simulink model "SolarSail"  (R2024a)
settings: Solver=ode3  StartTime=0.0  StopTime=2*24*60*60  FixedStep=30  MinStep=1  RelTol=1e-3
model workspace (MAT data in the model file):
  I_s = [344.15  0  0; 0  344.15  0; 0  0  688.24]
  LocalBodyOffset = [45 0 0]
undefined symbols (not defined in the file): IAU, juliandate, WMM2020
libraries: aerolibutil x15, matrix_library x14, simulink_extras x6, sharedtransform x5, aerolibtransform2 x4, aerolibconvert2 x4, aerolibatmos2 x1, aerolibsatdyn x1, aerolibobsolete x1, aerolibattitudesys x1, simulink x1, vrlib x1
(part 1 of 2)
settings Model: Creator=pierc  LastModifiedBy=pierc
settings SolverCC: InitialStep=1

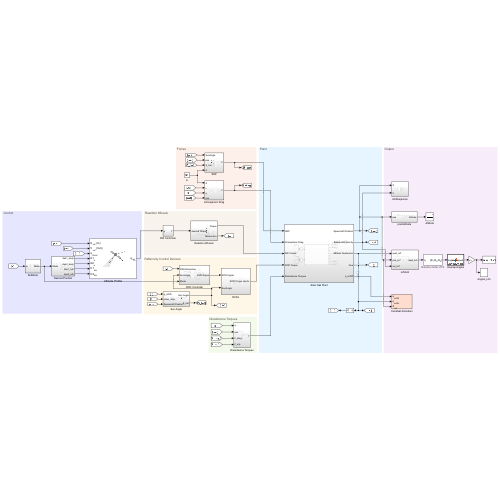
[thumbnail: Simulink's stored preview of the top-level diagram]
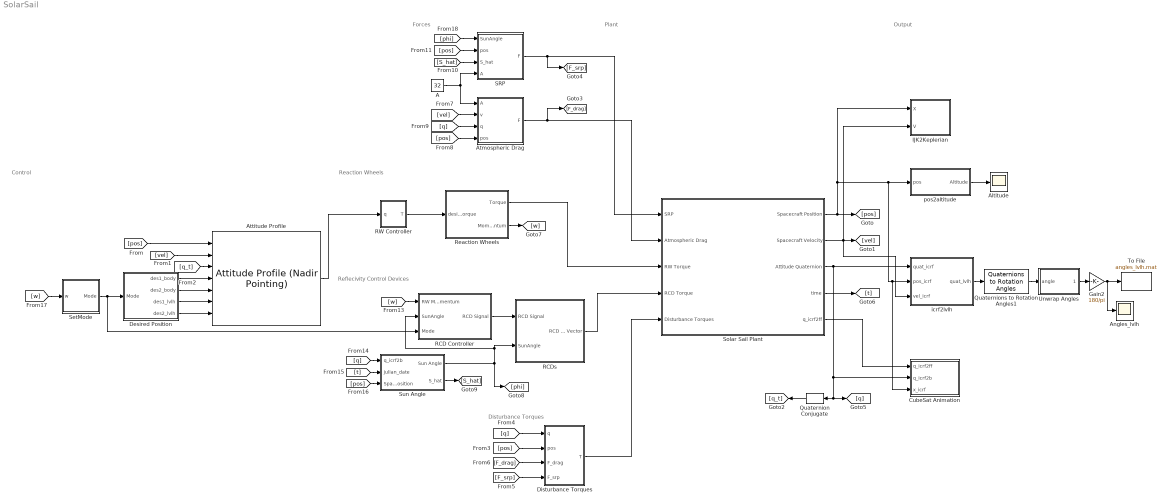
== system SolarSail ==
  note: Control
  note: Plant
  note: Reaction Wheels
  note: Disturbance Torques
  note: Forces
  note: Output
  note: Reflecivity Control Devices
  A : Constant  Value=32
  Altitude : Scope
  Angles_lvlh : Scope
  Atmospheric Drag : Subsystem
  "Attitude Profile " : aerolibsatdyn/Attitude Profile (Nadir Pointing)  outputError=on  outputFinalAttitude=off  portFrame=ICRF  pointingMode=Custom  celestialTarget=Sun  tunablePointing=off  primaryAlignmentSrc=Port  primaryAlignment=[0 0 1]  secondaryAlignmentSrc=Port  secondaryAlignment=[1 0 0]  constraintFrame=LVLH  primaryConstraintSrc=Port  primaryConstraint=[1 0 0]  secondaryConstraintSrc=Port  secondaryConstraint=[0 1 0]
  CubeSat Animation : Subsystem  mask(Simulink 3D Animation of CubeSat){enableVis=on, startDate=juliandate(2024, 7, 11, 2, 0, 0), visSampleTime=60, cubesatSize=2e5, showAntenna=on, antennaHeight=1e6, antennaHalfAngle=15}
      mask prompts: enableVis "spacecraft:cubesat:AnimEnableVis"; startDate "spacecraft:cubesat:StartDate"; visSampleTime "spacecraft:cubesat:AnimSampleTime"; cubesatSize "spacecraft:cubesat:MdlSize"; showAntenna "spacecraft:cubesat:ShowCone"; antennaHeight "spacecraft:cubesat:ConeHeight"; antennaHalfAngle "spacecraft:cubesat:ConeAngle"
      mask help: spacecraft:cubesat:VisBlockDesc
      settings: OpenFcn=|
      | if ~builtin('license','test','virtual_reality_toolbox')
      |     set_param(gcb, 'enableVis', 'off');
      | end
      | open_system(gcb,'mask');
      mask Callback enableVis:
      | if strcmp(get_param(gcb,'enableVis'), 'on')
      |     [licAvail, ~] = builtin('license','checkout','Virtual_Reality_Toolbox');
      |     if licAvail
      |         enable = repmat({'on'},7,1);
      |         set_param(gcb, 'Commented', 'off');
      |     else
      |         enable = repmat({'off'},7,1);
      |         set_param(gcb, 'Commented', 'on');
      |         set_param(gcb,'enableVis', 'off');
      |     end
      |     clear licAvail
      | else
      |     enable = repmat({'off'},7,1);
      |     set_param(gcb, 'Commented', 'on');
      | end
      | enable{1} = 'on';
      | set_param(gcb,'MaskEnables', enable);
      | clear enable
      mask Callback showAntenna:
      | if strcmp(get_param(gcb, 'enableVis'), 'on')
      |     enable = get_param(gcb,'MaskEnables');
      |     if strcmp(get_param(gcb, 'showAntenna'), 'off')
      |         enable(6:7) = {'off'};
      |     else
      |         enable(6:7) = {'on'};
      |     end
      |     set_param(gcb,'MaskEnables', enable);
      |     clear enable
      | end
      mask DialogControl enableVis Prompt: Enable visualization with Simulink 3D Animation
      mask DialogControl vrOpenBtn Prompt: spacecraft:cubesat:AnimOpenBtn
      mask DialogControl vrOpenBtn Callback:
      | if builtin('license','checkout','Virtual_Reality_Toolbox')
      |     vrmfunc('FnOpen',getSimulinkBlockHandle([gcb '/VR Sink']));
      | end
      mask DialogControl startDate Prompt: Start date [Julian date]:
      mask DialogControl startDate Tooltip: spacecraft:cubesat:StartDateTT
      mask DialogControl visSampleTime Prompt: Animation refresh rate:
      mask DialogControl visSampleTime Tooltip: spacecraft:cubesat:AnimSampleTimeTT
      mask DialogControl cubesatSize Prompt: CubeSat display size [m]:
      mask DialogControl cubesatSize Tooltip: spacecraft:cubesat:MdlSizeTT
      mask DialogControl Container3 Prompt: spacecraft:cubesat:AntennaPropArea
      mask DialogControl showAntenna Prompt: Show antenna cone in animation
      mask DialogControl showAntenna Tooltip: spacecraft:cubesat:ShowConeTT
      mask DialogControl antennaHeight Prompt: Antenna cone height [m]:
      mask DialogControl antennaHeight Tooltip: spacecraft:cubesat:ConeHeightTT
      mask DialogControl antennaHalfAngle Prompt: Antenna cone half angle [deg]:
      mask DialogControl antennaHalfAngle Tooltip: spacecraft:cubesat:ConeAngleTT
      mask Display:
      | port_label('input', 3, 'X_{icrf}','texmode','on')
      | port_label('input', 2, 'q_{icrf2b}','texmode','on')
      | port_label('input', 1, 'q_{icrf2ff}','texmode','on')
  Desired Position : Subsystem
  Disturbance Torques : Subsystem
  Gain2 : Gain  Gain=180/pi
  IJK2Keplerian : Subsystem
  Quaternion Conjugate : aerolibutil/Quaternion Conjugate
  Quaternions to Rotation Angles1 : sharedtransform/Quaternions to Rotation Angles  rotationOrder=ZYX  aMode=aMode
  RCD Controller : Subsystem
  RCDs : Subsystem
  RW Controller : Subsystem
  Reaction Wheels : Subsystem
  SRP : Subsystem
  SetMode : Subsystem
  Solar Sail Plant : Subsystem
  Sun Angle : Subsystem
  To File : ToFile  Filename=angles_lvlh.mat  MatrixName=angles_lvlh  SaveFormat=Timeseries
      settings: Decimation=2
  Unwrap Angles : MATLAB Function  TreatAsAtomicUnit=on  SystemSampleTime=30
  icrf2lvlh : Subsystem
  pos2altitude : Subsystem
  wires:
  Solar Sail Plant/1(Spacecraft Position) -> icrf2lvlh/2(pos_icrf), CubeSat Animation/3(x_icrf), pos2altitude/1(pos), IJK2Keplerian/1(X), [pos]
  Solar Sail Plant/3(Attitude Quaternion) -> icrf2lvlh/1(quat_icrf), [q], Quaternion Conjugate/1, CubeSat Animation/2(q_icrf2b)
  Solar Sail Plant/5(q_icrf2ff) -> CubeSat Animation/1(q_icrf2ff)
  Gain2/1 -> To File/1, Angles_lvlh/1
  [pos] -> "Attitude Profile "/1
  Solar Sail Plant/2(Spacecraft Velocity) -> IJK2Keplerian/2(V), [vel], icrf2lvlh/3(vel_icrf)
  Quaternion Conjugate/1 -> [q_t]
  [q_t] -> "Attitude Profile "/3
  icrf2lvlh/1(quat_lvlh) -> Quaternions to Rotation Angles1/1
  Desired Position/4(des2_lvlh) -> "Attitude Profile "/7
  "Attitude Profile "/1 -> RW Controller/1(q)
  Desired Position/1(des1_body) -> "Attitude Profile "/4
  Desired Position/2(des2_body) -> "Attitude Profile "/5
  Solar Sail Plant/4(time) -> [t]
  [vel] -> "Attitude Profile "/2
  RW Controller/1(T) -> Reaction Wheels/1(desired Torque)
  Reaction Wheels/1(Torque) -> Solar Sail Plant/3(RW Torque)
  pos2altitude/1(Altitude) -> Altitude/1
  [pos] -> Disturbance Torques/2(pos)
  [q] -> Disturbance Torques/1(q)
  Disturbance Torques/1(T) -> Solar Sail Plant/5(Disturbance Torques)
  [F_drag] -> Disturbance Torques/3(F_drag)
  [vel] -> Atmospheric Drag/2(v)
  [pos] -> Atmospheric Drag/4(pos)
  [q] -> Atmospheric Drag/3(q)
  Atmospheric Drag/1(F) -> [F_drag], Solar Sail Plant/2(Atmospheric Drag)
  [phi] -> SRP/1(SunAngle)
  A/1 -> Atmospheric Drag/1(A), SRP/4(A)
  SRP/1(F) -> [F_srp], Solar Sail Plant/1(SRP)
  [pos] -> Sun Angle/3(Spacecraft Position)
  [t] -> Sun Angle/2(julian_date)
  [q] -> Sun Angle/1(q_icrf2b)
  RCD Controller/1(RCD Signal) -> RCDs/1(RCD Signal)
  Sun Angle/1(Sun Angle) -> [phi], RCD Controller/2(SunAngle), RCDs/2(SunAngle)
  RCDs/1(RCD Torque Vector) -> Solar Sail Plant/4(RCD Torque)
  SetMode/1(Mode) -> RCD Controller/3(Mode), Desired Position/1(Mode)
  [w] -> RCD Controller/1(RW Momentum)
  Reaction Wheels/2(Momentum) -> [w]
  [w] -> SetMode/1(w)
  Desired Position/3(des1_lvlh) -> "Attitude Profile "/6
  Quaternions to Rotation Angles1/1 -> Unwrap Angles/1(angle)
  Unwrap Angles/1(unwrapped) -> Gain2/1
  [pos] -> SRP/2(pos)
  [F_srp] -> Disturbance Torques/4(F_srp)
  Sun Angle/2(S_hat) -> [S_hat]
  [S_hat] -> SRP/3(S_hat)

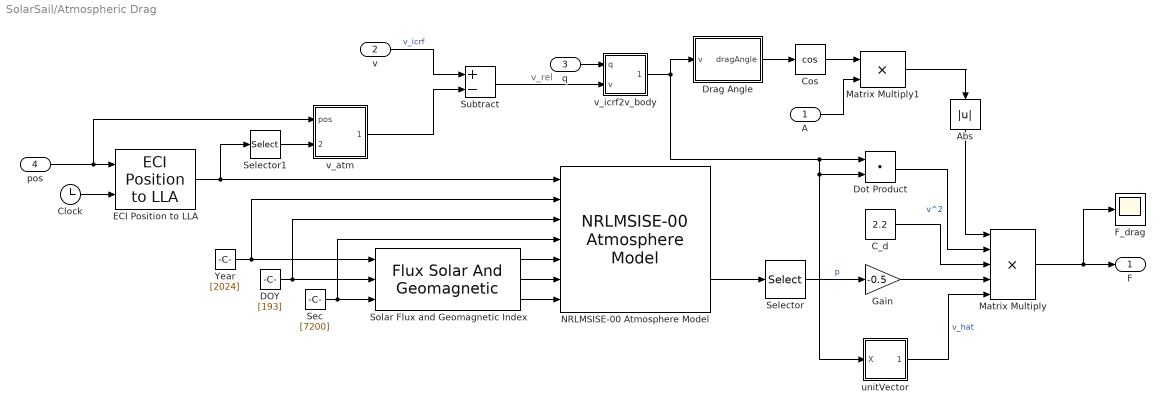
== system SolarSail/Atmospheric Drag ==
  note: v_rel
  A : Inport
  v : Inport  Port=2
  q : Inport  Port=3
  pos : Inport  Port=4
  Abs : Abs  SaturateOnIntegerOverflow=off
  C_d : Constant  Value=2.2
  Clock : Clock
  Cos : Trigonometry  Operator=cos
  DOY : Constant  Value=[193]
  Dot Product : DotProduct  OutDataTypeStr=Inherit: Inherit via internal rule
  Drag Angle : Subsystem
  ECI Position to LLA : aerolibtransform2/ECI Position to LLA  red=IAU-2000/2006  year=2024  month=July  day=11  hour=2  min=0  sec=0  deltaT=Sec  errorflag=Error  extraparamflag=off  eunits=Metric (MKS)  earthmodel=WGS84  flat=1/298.257223563  eqradius=6378137
      settings: AttributesFormatString=%<red>
  F_drag : Scope
  Gain : Gain  Gain=-0.5
  Matrix Multiply : Product  Inputs=5
  Matrix Multiply1 : Product
  NRLMSISE-00 Atmosphere Model : aerolibatmos2/NRLMSISE-00 Atmosphere Model  units=Metric (MKS)  lst_input=off  flux_ap_input=on  flags_input=Internal  flags=ones(1,23)  oxygen_in=on  action=Warning
  Sec : Constant  Value=[7200]
  Selector : Selector  InputPortWidth=9  IndexOptions=Index vector (dialog)  Indices=[6]  OutputSizes=1
  Selector1 : Selector  InputPortWidth=3  IndexOptions=Index vector (dialog)  Indices=[1]  OutputSizes=1
  Solar Flux and Geomagnetic Index : FluxSolarAndGeomagnetic
  Subtract : Sum  Inputs=+-
  Year : Constant  Value=[2024]
  unitVector : Subsystem
  v_atm : Subsystem
  v_icrf2v_body : Subsystem
  F : Outport
  wires:
  NRLMSISE-00 Atmosphere Model/2 -> Selector/1
  ECI Position to LLA/1 -> Selector1/1, NRLMSISE-00 Atmosphere Model/1
  pos/1 -> v_atm/1(pos), ECI Position to LLA/1
  DOY/1 -> NRLMSISE-00 Atmosphere Model/3, Solar Flux and Geomagnetic Index/2
  Solar Flux and Geomagnetic Index/3 -> NRLMSISE-00 Atmosphere Model/7
  Solar Flux and Geomagnetic Index/2 -> NRLMSISE-00 Atmosphere Model/6
  Clock/1 -> ECI Position to LLA/2
  Solar Flux and Geomagnetic Index/1 -> NRLMSISE-00 Atmosphere Model/5
  Gain/1 -> Matrix Multiply/4
  Selector/1 -> Gain/1  "p"
  Cos/1 -> Matrix Multiply1/1
  Drag Angle/1(dragAngle) -> Cos/1
  C_d/1 -> Matrix Multiply/3
  Matrix Multiply1/1 -> Abs/1
  Year/1 -> NRLMSISE-00 Atmosphere Model/2, Solar Flux and Geomagnetic Index/1
  Sec/1 -> NRLMSISE-00 Atmosphere Model/4, Solar Flux and Geomagnetic Index/3
  A/1 -> Matrix Multiply1/2
  Dot Product/1 -> Matrix Multiply/2  "v^2"
  Selector1/1 -> v_atm/2(latitude)
  v_atm/1(v_atm) -> Subtract/2
  Subtract/1 -> v_icrf2v_body/2(v)
  v/1 -> Subtract/1  "v_icrf"
  v_icrf2v_body/1(v_body) -> unitVector/1(X), Dot Product/2, Dot Product/1, Drag Angle/1(v)
  q/1 -> v_icrf2v_body/1(q)
  Matrix Multiply/1 -> F_drag/1, F/1
  Abs/1 -> Matrix Multiply/1
  unitVector/1(X_hat) -> Matrix Multiply/5  "v_hat"

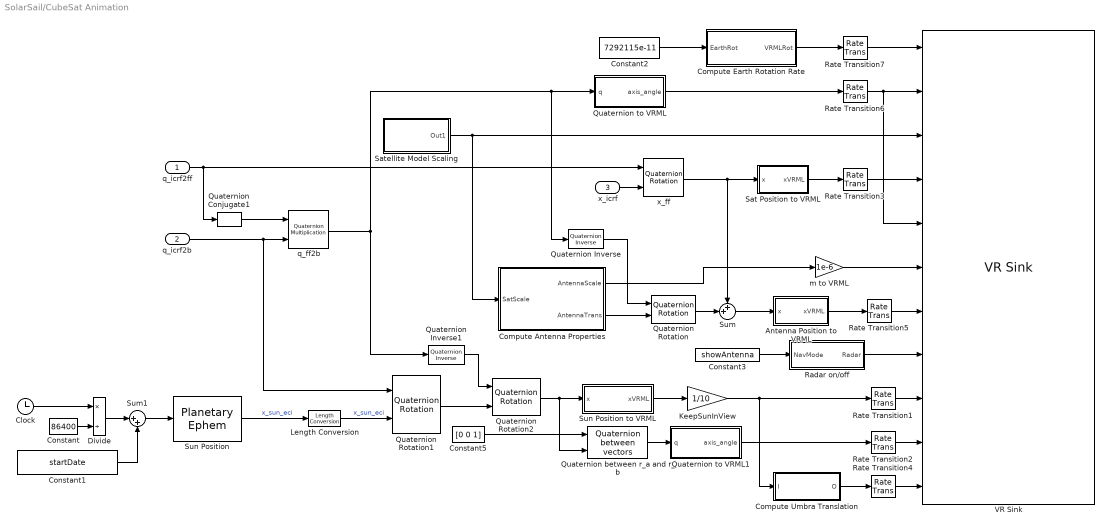
== system SolarSail/CubeSat Animation ==
  q_icrf2ff : Inport  PortDimensions=4
  q_icrf2b : Inport  Port=2  PortDimensions=4
  x_icrf : Inport  Port=3  PortDimensions=3
  Antenna Position to VRML : Subsystem
  Clock : Clock
  Compute Antenna Properties : Subsystem
  Compute Earth Rotation Rate : Subsystem
  Compute Umbra Translation : Subsystem
  Constant : Constant  Value=86400
  Constant1 : Constant  Value=startDate  SampleTime=visSampleTime
  Constant2 : Constant  Value=7292115e-11
  Constant3 : Constant  Value=showAntenna
  Constant5 : Constant  Value=[0 0 1]
  Divide : Product  Inputs=*/
  KeepSunInView : Gain  Gain=1/10
  Length Conversion : aerolibconvert2/Length Conversion  IU=km  OU=m
  Quaternion Conjugate1 : aerolibutil/Quaternion Conjugate
  Quaternion Inverse : aerolibutil/Quaternion Inverse
  Quaternion Inverse1 : aerolibutil/Quaternion Inverse
  Quaternion Rotation : aerolibutil/Quaternion Rotation
  Quaternion Rotation1 : aerolibutil/Quaternion Rotation
  Quaternion Rotation2 : aerolibutil/Quaternion Rotation
  Quaternion between r_a and r_b : aerolibattitudesys/Quaternion between vectors
  Quaternion to VRML : Subsystem
  Quaternion to VRML1 : Subsystem
  Radar on/off : Subsystem
  Rate Transition{1..7} (7 alike) : RateTransition
  Sat Position to VRML : Subsystem
  Satellite Model Scaling : Subsystem
  Sum : Sum  Inputs=++|
  Sum1 : Sum  Inputs=|++
  Sun Position : PlanetaryEphem  ephemerisModel=DE421  target=Sun  outputVelocity=off
  Sun Position to VRML : Subsystem
  VR Sink : vrlib/VR Sink  InstantiateOnLoad=on  SampleTime=visSampleTime  ViewEnable=on  RemoteChange=off  RemoteView=off  FieldsWritten=Earth.rotation.4.1.1.double#Satellite.rotation.4.1.1.double#Satellite.scale.3.1.1.double#Satellite.translation.3.1.1.double#AntennaCone.rotation.4.1.1.double#AntennaCone.scale.3.1.1.double#AntennaCone.translation.3.1.1.double#AntennaMaterial.transparency.1.1.1.double#Sun.translation.3.1.1.double#Umbra.rotation.4.1.1.double#Umbra.translation.3.1.1.double  WorldFileName=cubesatAnim.wrl  WorldDescription=CubeSat Orbit Animation  AutoView=off  VideoDimensions=[]  AllowVariableSize=off
  m to VRML : Gain  Gain=1e-6
  q_ff2b : aerolibutil/Quaternion Multiplication
  x_ff : aerolibutil/Quaternion Rotation
  wires:
  Quaternion to VRML1/1(axis_angle) -> Rate Transition2/1
  Quaternion between r_a and r_b/1 -> Quaternion to VRML1/1(q)
  Constant2/1 -> Compute Earth Rotation Rate/1(EarthRot)
  Compute Antenna Properties/1(AntennaScale) -> m to VRML/1
  Quaternion to VRML/1(axis_angle) -> Rate Transition6/1
  Compute Umbra Translation/1(O) -> Rate Transition4/1
  q_icrf2b/1 -> Quaternion Rotation1/1, q_ff2b/2
  Quaternion Rotation2/1 -> Sun Position to VRML/1(x), Quaternion between r_a and r_b/2
  Constant5/1 -> Quaternion between r_a and r_b/1
  KeepSunInView/1 -> Compute Umbra Translation/1(I), Rate Transition1/1
  Sun Position to VRML/1(xVRML) -> KeepSunInView/1
  Sat Position to VRML/1(xVRML) -> Rate Transition3/1
  Compute Antenna Properties/2(AntennaTrans) -> Quaternion Rotation/2
  Satellite Model Scaling/1(Out1) -> VR Sink/3, Compute Antenna Properties/1(SatScale)
  Constant3/1 -> Radar on/off/1(NavMode)
  q_ff2b/1 -> Quaternion Inverse/1, Quaternion to VRML/1(q), Quaternion Inverse1/1
  Quaternion Rotation1/1 -> Quaternion Rotation2/2
  Compute Earth Rotation Rate/1(VRMLRot) -> Rate Transition7/1
  Antenna Position to VRML/1(xVRML) -> Rate Transition5/1
  Quaternion Inverse/1 -> Quaternion Rotation/1
  x_ff/1 -> Sum/1, Sat Position to VRML/1(x)
  Quaternion Rotation/1 -> Sum/2
  Sum/1 -> Antenna Position to VRML/1(x)
  Quaternion Inverse1/1 -> Quaternion Rotation2/1
  Rate Transition4/1 -> VR Sink/11
  Rate Transition2/1 -> VR Sink/10
  Rate Transition1/1 -> VR Sink/9
  Rate Transition5/1 -> VR Sink/7
  m to VRML/1 -> VR Sink/6
  Rate Transition3/1 -> VR Sink/4
  Rate Transition7/1 -> VR Sink/1
  Rate Transition6/1 -> VR Sink/5, VR Sink/2
  Constant1/1 -> Sum1/2
  Divide/1 -> Sum1/1
  Constant/1 -> Divide/2
  Sun Position/1 -> Length Conversion/1  "x_sun_eci"
  Clock/1 -> Divide/1
  Length Conversion/1 -> Quaternion Rotation1/2  "x_sun_eci"
  Sum1/1 -> Sun Position/1
  Radar on/off/1(Radar) -> VR Sink/8
  Quaternion Conjugate1/1 -> q_ff2b/1
  q_icrf2ff/1 -> Quaternion Conjugate1/1, x_ff/1
  x_icrf/1 -> x_ff/2

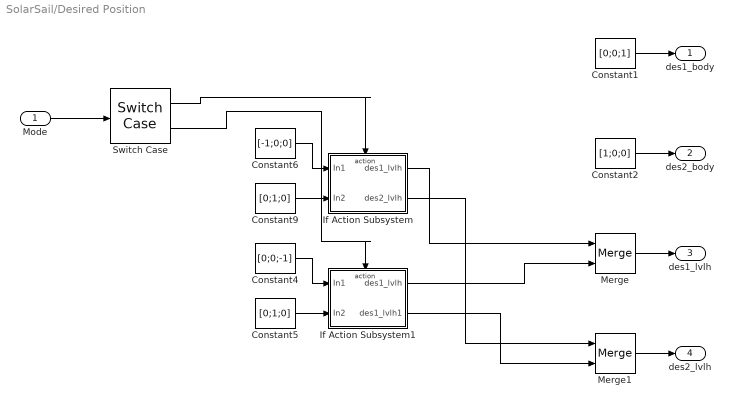
== system SolarSail/Desired Position ==
  Mode : Inport
  Constant1 : Constant  Value=[0;0;1]
  Constant2 : Constant  Value=[1;0;0]
  Constant4 : Constant  Value=[0;0;-1]
  Constant5 : Constant  Value=[0;1;0]
  Constant6 : Constant  Value=[-1;0;0]
  Constant9 : Constant  Value=[0;1;0]
  If Action Subsystem : Subsystem  TreatAsAtomicUnit=on
  If Action Subsystem1 : Subsystem  TreatAsAtomicUnit=on
  Merge : Merge
  Merge1 : Merge
  Switch Case : SwitchCase  CaseConditions={0,1}  ShowDefaultCase=off
  des1_body : Outport
  des2_body : Outport  Port=2
  des1_lvlh : Outport  Port=3
  des2_lvlh : Outport  Port=4
  wires:
  Constant1/1 -> des1_body/1
  Constant2/1 -> des2_body/1
  Mode/1 -> Switch Case/1
  Switch Case/1 -> If Action Subsystem/Action
  Constant6/1 -> If Action Subsystem/1(In1)
  Constant9/1 -> If Action Subsystem/2(In2)
  Switch Case/2 -> If Action Subsystem1/Action
  Constant4/1 -> If Action Subsystem1/1(In1)
  Constant5/1 -> If Action Subsystem1/2(In2)
  Merge/1 -> des1_lvlh/1
  Merge1/1 -> des2_lvlh/1
  If Action Subsystem/1(des1_lvlh) -> Merge/1
  If Action Subsystem1/1(des1_lvlh) -> Merge/2
  If Action Subsystem/2(des2_lvlh) -> Merge1/1
  If Action Subsystem1/2(des1_lvlh1) -> Merge1/2

== system SolarSail/Disturbance Torques ==
  q : Inport
  pos : Inport  Port=2
  F_drag : Inport  Port=3
  F_srp : Inport  Port=4
  Add : Sum  Inputs=+++
  Atmospheric Drag Torque : Subsystem
  Magnetic Field Torque : Subsystem
  SRP Torque : Subsystem
  T : Outport
  wires:
  pos/1 -> Magnetic Field Torque/1(pos)
  q/1 -> Magnetic Field Torque/2(q)
  Add/1 -> T/1  "T"
  F_drag/1 -> Atmospheric Drag Torque/1(F_drag)
  Atmospheric Drag Torque/1(T) -> Add/2
  SRP Torque/1(T) -> Add/1
  Magnetic Field Torque/1(T) -> Add/3
  F_srp/1 -> SRP Torque/1(F_srp)

== system SolarSail/IJK2Keplerian ==
  X : Inport
  V : Inport  Port=2
  Bus Creator : BusCreator  Inputs=6
  MATLAB Function : MATLAB Function  TreatAsAtomicUnit=on
  To Workspace : ToWorkspace  VariableName=OrbitalElements  SaveFormat=Timeseries  SampleTime=-1
  wires:
  X/1 -> MATLAB Function/1(r_ijk)
  V/1 -> MATLAB Function/2(v_ijk)
  MATLAB Function/1(a) -> Bus Creator/1
  MATLAB Function/2(ecc) -> Bus Creator/2
  MATLAB Function/3(incl) -> Bus Creator/3
  MATLAB Function/4(RAAN) -> Bus Creator/4
  MATLAB Function/5(argp) -> Bus Creator/5
  MATLAB Function/6(nu) -> Bus Creator/6
  Bus Creator/1 -> To Workspace/1

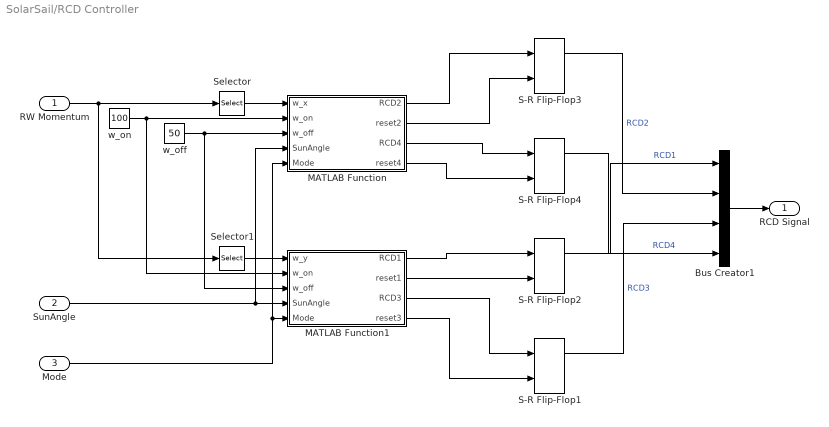
== system SolarSail/RCD Controller ==
  RW Momentum : Inport
  SunAngle : Inport  Port=2
  Mode : Inport  Port=3
  Bus Creator1 : BusCreator  Inputs=4
  MATLAB Function : MATLAB Function  TreatAsAtomicUnit=on
  MATLAB Function1 : MATLAB Function  TreatAsAtomicUnit=on
  S-R Flip-Flop{1..4} (4 alike) : simulink_extras/Flip Flops/S-R Flip-Flop  initial_condition=0
  Selector : Selector  InputPortWidth=3  IndexOptions=Index vector (dialog)  Indices=[1]  OutputSizes=1
  Selector1 : Selector  InputPortWidth=3  IndexOptions=Index vector (dialog)  Indices=[2]  OutputSizes=1
  w_off : Constant  Value=50
  w_on : Constant  Value=100
  RCD Signal : Outport
  wires:
  Bus Creator1/1 -> RCD Signal/1
  MATLAB Function1/1(RCD1) -> S-R Flip-Flop2/1
  MATLAB Function1/2(reset1) -> S-R Flip-Flop2/2
  MATLAB Function1/3(RCD3) -> S-R Flip-Flop1/1
  MATLAB Function1/4(reset3) -> S-R Flip-Flop1/2
  S-R Flip-Flop1/1 -> Bus Creator1/3  "RCD3"
  S-R Flip-Flop2/1 -> Bus Creator1/1  "RCD1"
  w_off/1 -> MATLAB Function1/3(w_off), MATLAB Function/3(w_off)
  w_on/1 -> MATLAB Function1/2(w_on), MATLAB Function/2(w_on)
  MATLAB Function/1(RCD2) -> S-R Flip-Flop3/1
  MATLAB Function/2(reset2) -> S-R Flip-Flop3/2
  MATLAB Function/3(RCD4) -> S-R Flip-Flop4/1
  MATLAB Function/4(reset4) -> S-R Flip-Flop4/2
  S-R Flip-Flop4/1 -> Bus Creator1/4  "RCD4"
  S-R Flip-Flop3/1 -> Bus Creator1/2  "RCD2"
  Selector/1 -> MATLAB Function/1(w_x)
  RW Momentum/1 -> Selector/1, Selector1/1
  Selector1/1 -> MATLAB Function1/1(w_y)
  SunAngle/1 -> MATLAB Function/4(SunAngle), MATLAB Function1/4(SunAngle)
  Mode/1 -> MATLAB Function/5(Mode), MATLAB Function1/5(Mode)

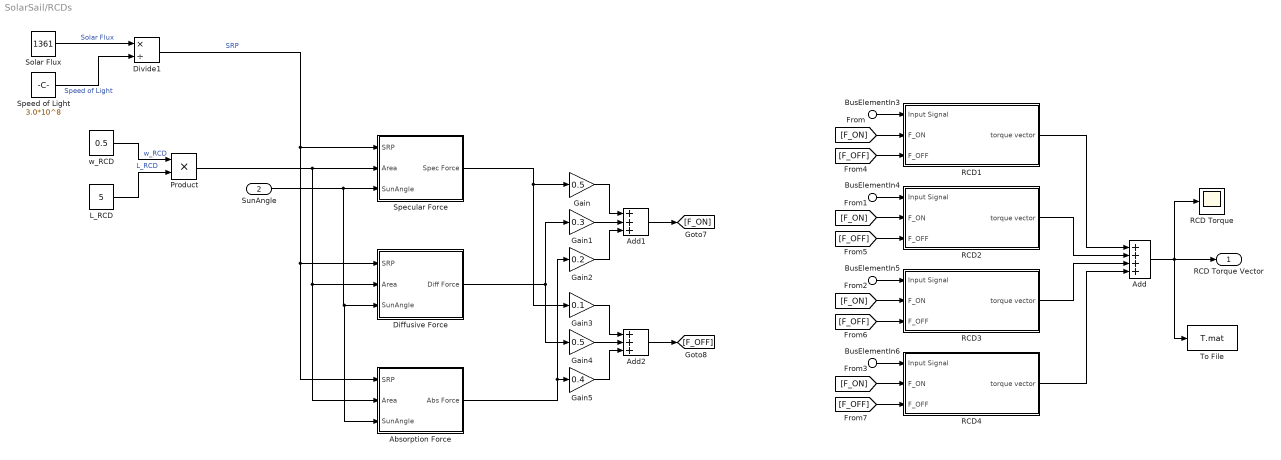
== system SolarSail/RCDs ==
  BusElementIn3 : Inport  PortName=RCD Signal  Element=RCD1
  BusElementIn4 : Inport  PortName=RCD Signal  Element=RCD2
  BusElementIn5 : Inport  PortName=RCD Signal  Element=RCD3
  BusElementIn6 : Inport  PortName=RCD Signal  Element=RCD4
  SunAngle : Inport  Port=2
  Absorption Force : Subsystem
  Add : Sum  Inputs=++++
  Add1 : Sum  Inputs=+++
  Add2 : Sum  Inputs=+++
  Diffusive Force : Subsystem
  Divide1 : Product  Inputs=*/
  Gain : Gain  Gain=0.5
  Gain1 : Gain  Gain=0.3
  Gain2 : Gain  Gain=0.2
  Gain3 : Gain  Gain=0.1
  Gain4 : Gain  Gain=0.5
  Gain5 : Gain  Gain=0.4
  L_RCD : Constant  Value=5
  Product : Product
  RCD Torque : Scope
  RCD1 : Subsystem
  RCD2 : Subsystem
  RCD3 : Subsystem
  RCD4 : Subsystem
  Solar Flux : Constant  Value=1361
  Specular Force : Subsystem
  Speed of Light : Constant  Value=3.0*10^8
  To File : ToFile  Filename=T.mat  MatrixName=T  SaveFormat=Timeseries
      settings: Decimation=2
  w_RCD : Constant  Value=0.5
  RCD Torque Vector : Outport
  wires:
  RCD2/1(torque vector) -> Add/2
  RCD1/1(torque vector) -> Add/1
  RCD4/1(torque vector) -> Add/4
  RCD3/1(torque vector) -> Add/3
  Add/1 -> To File/1, RCD Torque/1, RCD Torque Vector/1
  BusElementIn3/1 -> RCD1/1(Input Signal)
  BusElementIn4/1 -> RCD2/1(Input Signal)
  BusElementIn5/1 -> RCD3/1(Input Signal)
  [F_ON] -> RCD1/2(F_ON)
  [F_ON] -> RCD2/2(F_ON)
  [F_ON] -> RCD3/2(F_ON)
  [F_ON] -> RCD4/2(F_ON)
  [F_OFF] -> RCD1/3(F_OFF)
  [F_OFF] -> RCD2/3(F_OFF)
  [F_OFF] -> RCD3/3(F_OFF)
  [F_OFF] -> RCD4/3(F_OFF)
  BusElementIn6/1 -> RCD4/1(Input Signal)
  Speed of Light/1 -> Divide1/2  "Speed of Light"
  Solar Flux/1 -> Divide1/1  "Solar Flux"
  L_RCD/1 -> Product/2  "L_RCD"
  Divide1/1 -> Absorption Force/1(SRP), Diffusive Force/1(SRP), Specular Force/1(SRP)  "SRP"
  w_RCD/1 -> Product/1  "w_RCD"
  Add1/1 -> [F_ON]
  Gain/1 -> Add1/1
  Gain1/1 -> Add1/2
  Gain2/1 -> Add1/3
  Gain5/1 -> Add2/3
  Gain3/1 -> Add2/1
  Add2/1 -> [F_OFF]
  Gain4/1 -> Add2/2
  Diffusive Force/1(Diff Force) -> Gain1/1, Gain4/1
  Absorption Force/1(Abs Force) -> Gain2/1, Gain5/1
  Specular Force/1(Spec Force) -> Gain3/1, Gain/1
  SunAngle/1 -> Absorption Force/3(SunAngle), Diffusive Force/3(SunAngle), Specular Force/3(SunAngle)
  Product/1 -> Absorption Force/2(Area), Diffusive Force/2(Area), Specular Force/2(Area)

== system SolarSail/RW Controller ==
  q : Inport
  D Lookup : Lookup_n-D  NumberOfTableDimensions=1  BreakpointsSpecification=Even spacing  BreakpointsForDimension1=[-5:5]  BreakpointsForDimension1FirstPoint=0.0075  BreakpointsForDimension1Spacing=0.02  Table=[0.04;0.03]  ExtrapMethod=Clip  UseLastTableValue=on  InternalRulePriority=Speed  RndMeth=Simplest
  Demo Controller : slpidlib/PID Controller  Controller=PD  Form=Parallel  TimeDomain=Discrete-time  UseExternalTs=off  SampleTime=-1  IntegratorMethod=Trapezoidal  FilterMethod=Trapezoidal  ControllerParametersSource=external  P=.0002  I=.0000002  UseKiTs=off  D=.025  UseExternalDerivativeSource=off  N=1  UseFilter=off  TunerSelectOption=Transfer Function Based (PID Tuner App)  InitialConditionSource=internal  InitialConditionForIntegrator=0  InitialConditionForFilter=0  DifferentiatorICPrevScaledInput=0  ExternalReset=none  TrackingMode=off  Kt=1  LimitOutput=on  SatLimitsSource=internal  UpperSaturationLimit=0.008  LowerSaturationLimit=-0.008  LinearizeAsGain=on  AntiWindupMode=none  Kb=1  LimitIntegrator=off  UpperIntegratorSaturationLimit=inf  LowerIntegratorSaturationLimit=-inf  POutMin=[]  POutMax=[]  IOutMin=[]  IOutMax=[]  DOutMin=[]  DOutMax=[]  NOutMin=[]  NOutMax=[]  SumOutMin=[]  SumOutMax=[]  SaturationOutMin=[]  SaturationOutMax=[]  PParamMin=[]  PParamMax=[]  IParamMin=[]  IParamMax=[]  DParamMin=[]  DParamMax=[]  NParamMin=[]  NParamMax=[]  KbParamMin=[]  KbParamMax=[]  KtParamMin=[]  KtParamMax=[]  KbOutMin=[]  KbOutMax=[]  KtOutMin=[]  KtOutMax=[]  IntegratorOutMin=[]  IntegratorOutMax=[]  FilterOutMin=[]  FilterOutMax=[]  SumI1OutMin=[]  SumI1OutMax=[]  SumI2OutMin=[]  SumI2OutMax=[]  SumI3OutMin=[]  SumI3OutMax=[]  SumI4OutMin=[]  SumI4OutMax=[]  SumDOutMin=[]  SumDOutMax=[]  DifferentiatorOutMin=[]  DifferentiatorOutMax=[]  FilterDiffOutCoefMin=[]  FilterDiffOutCoefMax=[]  ReciprocalOutMin=[]  ReciprocalOutMax=[]  SumDenOutMin=[]  SumDenOutMax=[]  SumNumOutMin=[]  SumNumOutMax=[]  DivideOutMin=[]  DivideOutMax=[]  UdiffTsProdOutMin=[]  UdiffTsProdOutMax=[]  NTsProdOutMin=[]  NTsProdOutMax=[]  UintegralTsProdOutMin=[]  UintegralTsProdOutMax=[]  UngainTsProdOutMin=[]  UngainTsProdOutMax=[]  ClampingZeroOutDataTypeStr=Inherit: Inherit via back propagation  ClampingZeroOutMin=[]  ClampingZeroOutMax=[]  FilterDenConstantOutDataTypeStr=Inherit: Inherit via back propagation  FilterDenConstantOutMin=[]  FilterDenConstantOutMax=[]  PCopyOutDataTypeStr=Inherit: Inherit via back propagation  PCopyOutMin=[]  PCopyOutMax=[]  NCopyOutDataTypeStr=Inherit: Inherit via back propagation  NCopyOutMin=[]  NCopyOutMax=[]  IntegratorContinuousStateAttributes=''  IntegratorStateMustResolveToSignalObject=off  IntegratorRTWStateStorageClass=Auto  FilterContinuousStateAttributes=''  FilterStateMustResolveToSignalObject=off  FilterRTWStateStorageClass=Auto  ParallelPVariant=ExternalParameters  IdealPVariant=Disabled  IVariant=Disabled  DVariant=ExternalParameters  IntegratorVariant=Disabled  SatVariant=Enabled  AWVariant=Disabled  PCopyVariant=Disabled  TRVariant=Disabled  FdbkBlocksVariant=Forward  IdealPFdbkVariant=Disabled  SatFdbkVariant=Disabled  DerivativeFilterVariant=Differentiator  NVariant=Passthrough  NCopyVariant=Disabled_SignalSpec  FilterICVariant=InternalICsDifferentiator  IntegratorICVariant=Disabled  ExternalResetVariant=Disabled  TRSumVariant=Passthrough  SumFdbkVariant=Disabled  SumVariant=Sum_PD  TsampFilterVariant=InternalTs  TsampNgainVariant=Passthrough  TsampIntegralVariant=Disabled_SignalSpec  ExternalSaturationOutDataTypeStr=Inherit: Same as second input  DerivativeSourceVariant=ErrorSignal
  Dot Product : DotProduct  OutDataTypeStr=Inherit: Inherit via internal rule
  Error : Scope
  P : Scope
  P Lookup : Lookup_n-D  NumberOfTableDimensions=1  BreakpointsSpecification=Even spacing  BreakpointsForDimension1=[-5:5]  BreakpointsForDimension1FirstPoint=0.0075  BreakpointsForDimension1Spacing=0.02  Table=[0.0004;0.00006]  ExtrapMethod=Clip  UseLastTableValue=on  InternalRulePriority=Speed  RndMeth=Simplest
  Quaternions to Rotation Angles : sharedtransform/Quaternions to Rotation Angles  rotationOrder=XYZ  aMode=aMode
  Saturation : Saturate  UpperLimit=0.001  LowerLimit=-0.001
  T : Outport
  wires:
  q/1 -> Quaternions to Rotation Angles/1
  Quaternions to Rotation Angles/1 -> Error/1, Demo Controller/1, Dot Product/2, Dot Product/1
  Demo Controller/1 -> Saturation/1
  Saturation/1 -> T/1
  Dot Product/1 -> D Lookup/1, P Lookup/1
  P Lookup/1 -> Demo Controller/2, P/1
  D Lookup/1 -> Demo Controller/3

== system SolarSail/Reaction Wheels ==
  desired Torque : Inport
  I_w : Constant  Value=1.112*10^-4
  Memory1 : Memory
  Saturation : Saturate  UpperLimit=1017  LowerLimit=-1017
  T : Scope
  T to w : Subsystem
  To File : ToFile  Filename=w.mat  MatrixName=w  SaveFormat=Timeseries
  deltaT : Subsystem
  w : Scope
  w to T : Subsystem
  Torque : Outport
  Momentum : Outport  Port=2
  wires:
  Saturation/1 -> To File/1, w/1, w to T/1(w_f), Memory1/1, Momentum/1
  Memory1/1 -> w to T/2(w_i), T to w/1(w_prev)
  I_w/1 -> w to T/3(I), T to w/3(I)
  T to w/1(w) -> Saturation/1
  deltaT/1(dT) -> T to w/4(dT), w to T/4(dT)
  desired Torque/1 -> T to w/2(T)
  w to T/1(T) -> Torque/1, T/1

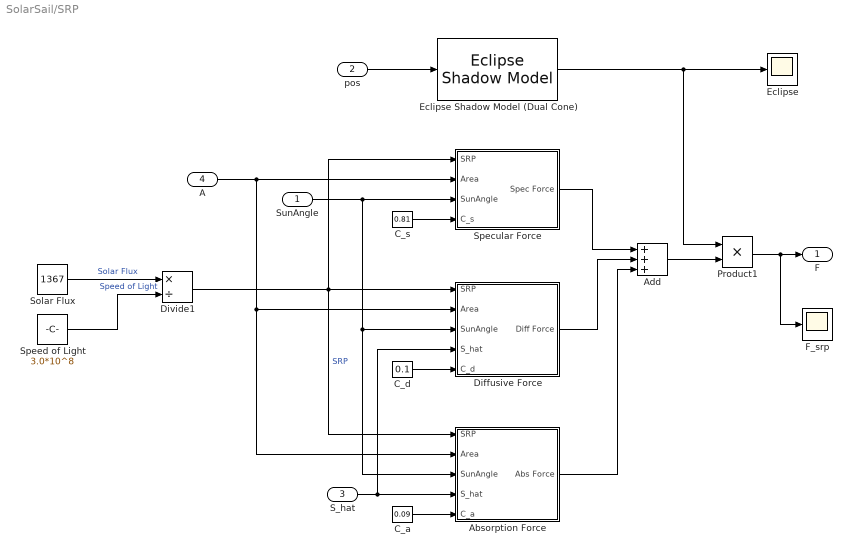
== system SolarSail/SRP ==
  SunAngle : Inport
  pos : Inport  Port=2
  S_hat : Inport  Port=3
  A : Inport  Port=4
  Absorption Force : Subsystem
  Add : Sum  Inputs=+++
  C_a : Constant  Value=0.09
  C_d : Constant  Value=0.1
  C_s : Constant  Value=0.81
  Diffusive Force : Subsystem
  Divide1 : Product  Inputs=*/
  Eclipse : Scope
  Eclipse Shadow Model (Dual Cone) : EclipseShadowModel  startDate=juliandate(2024, 7, 11,2,0,0)  ephemerisModel=DE432t  ephemerisStartDate=juliandate(2024, 7, 11,2,0,0)  ephemerisEndDate=juliandate(2024, 7, 12,2,0,0)
  F_srp : Scope
  Product1 : Product
  Solar Flux : Constant  Value=1367
  Specular Force : Subsystem
  Speed of Light : Constant  Value=3.0*10^8
  F : Outport
  wires:
  Solar Flux/1 -> Divide1/1  "Solar Flux"
  Speed of Light/1 -> Divide1/2  "Speed of Light"
  pos/1 -> Eclipse Shadow Model (Dual Cone)/1
  Eclipse Shadow Model (Dual Cone)/1 -> Product1/1, Eclipse/1
  Divide1/1 -> Absorption Force/1(SRP), Specular Force/1(SRP), Diffusive Force/1(SRP)  "SRP"
  SunAngle/1 -> Absorption Force/3(SunAngle), Diffusive Force/3(SunAngle), Specular Force/3(SunAngle)
  A/1 -> Absorption Force/2(Area), Diffusive Force/2(Area), Specular Force/2(Area)
  Specular Force/1(Spec Force) -> Add/1
  Diffusive Force/1(Diff Force) -> Add/2
  Add/1 -> Product1/2
  Product1/1 -> F_srp/1, F/1
  C_s/1 -> Specular Force/4(C_s)
  C_d/1 -> Diffusive Force/5(C_d)
  S_hat/1 -> Absorption Force/4(S_hat), Diffusive Force/4(S_hat)
  C_a/1 -> Absorption Force/5(C_a)
  Absorption Force/1(Abs Force) -> Add/3

== system SolarSail/SetMode ==
  w : Inport
  Cast To Double : DataTypeConversion  OutDataTypeStr=double  SaturateOnIntegerOverflow=off  RndMeth=Floor
  MATLAB Function : MATLAB Function  TreatAsAtomicUnit=on
  S-R Flip-Flop : simulink_extras/Flip Flops/S-R Flip-Flop  initial_condition=0
  Scope : Scope
  To File : ToFile  Filename=Mode.mat  MatrixName=Mode  SaveFormat=Timeseries
  Unit Delay : UnitDelay  SampleTime=-1  HasFrameUpgradeWarning=on
  w_off : Constant  Value=100
  w_on : Constant  Value=700
  Mode : Outport
  wires:
  w/1 -> Unit Delay/1
  Unit Delay/1 -> MATLAB Function/1(w)
  w_on/1 -> MATLAB Function/2(w_on)
  w_off/1 -> MATLAB Function/3(w_off)
  MATLAB Function/2(reset) -> S-R Flip-Flop/2
  MATLAB Function/1(Mode) -> S-R Flip-Flop/1
  S-R Flip-Flop/1 -> Cast To Double/1
  Cast To Double/1 -> To File/1, Mode/1, Scope/1

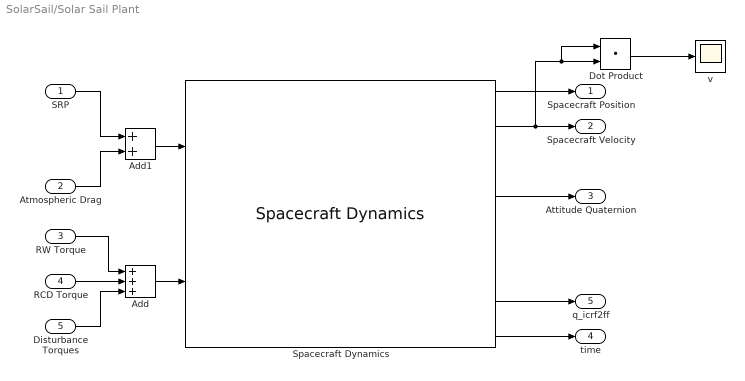
== system SolarSail/Solar Sail Plant ==
  SRP : Inport
  Atmospheric Drag : Inport  Port=2
  RW Torque : Inport  Port=3
  RCD Torque : Inport  Port=4
  Disturbance Torques : Inport  Port=5
  Add : Sum  Inputs=+++
  Add1 : Sum
  Dot Product : DotProduct  OutDataTypeStr=Inherit: Inherit via internal rule
  Spacecraft Dynamics : SpacecraftDynamics  outputAccel=on  startDate=juliandate(2024, 7, 11, 2, 0, 0)  mass=4.93  inertia=[3.79,-1.90*10^-4,-8.18*10^-4;-1.90*10^-4,3.79,1.47*10^-3;-8.18*10^-4,1.47*10^-3,7.33]  semiMajorAxis=7078140  eccentricity=0.001  inclination=98.1928  raan=22  argPeriapsis=360  trueAnomaly=0  attitude=[0.702,0.1842,-0.6827,0.085]  attitudeRate=[0, -0.06, 0]  outputAngAccel=on  outputTransform=on  ephemerisModel=DE432t  ephemerisStartDate=juliandate(2024, 7, 11, 2, 0, 0)  ephemerisEndDate=juliandate(2025, 1, 1, 0, 0, 0)  useThirdBodyGravity=on  srpArea=32
  v : Scope
  Spacecraft Position : Outport
  Spacecraft Velocity : Outport  Port=2
  Attitude Quaternion : Outport  Port=3
  time : Outport  Port=4
  q_icrf2ff : Outport  Port=5
  wires:
  Spacecraft Dynamics/1 -> Spacecraft Position/1
  Spacecraft Dynamics/4 -> Attitude Quaternion/1
  Spacecraft Dynamics/8 -> time/1
  Spacecraft Dynamics/7 -> q_icrf2ff/1
  RW Torque/1 -> Add/1
  Add/1 -> Spacecraft Dynamics/2
  Disturbance Torques/1 -> Add/3
  Add1/1 -> Spacecraft Dynamics/1
  SRP/1 -> Add1/1
  Atmospheric Drag/1 -> Add1/2
  RCD Torque/1 -> Add/2
  Spacecraft Dynamics/2 -> Dot Product/1, Dot Product/2, Spacecraft Velocity/1
  Dot Product/1 -> v/1

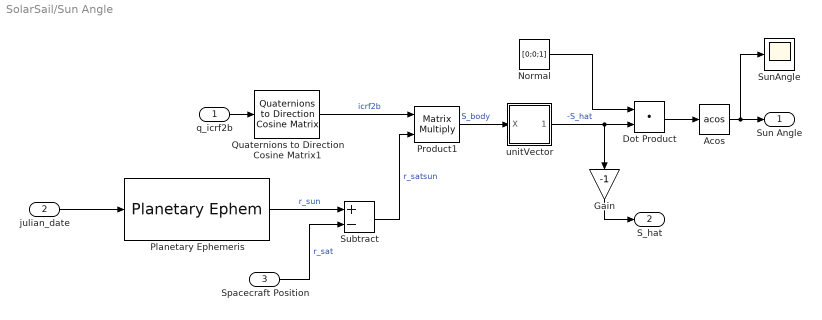
== system SolarSail/Sun Angle ==
  q_icrf2b : Inport
  julian_date : Inport  Port=2
  Spacecraft Position : Inport  Port=3
  Acos : Trigonometry  Operator=acos
  Dot Product : DotProduct  OutDataTypeStr=Inherit: Inherit via internal rule
  Gain : Gain  Gain=-1
  Normal : Constant  Value=[0;0;1]
  Planetary Ephemeris : PlanetaryEphem  units=m,m/s  ephemerisModel=DE432t  target=Sun  outputVelocity=off
  Product1 : Product  Multiplication=Matrix(*)
  Quaternions to Direction Cosine Matrix1 : sharedtransform/Quaternions to  Direction Cosine Matrix  aMode=aMode
      settings: LibrarySourceBlock=|
      | aerolibtransform2/Quaternions to
      | Direction Cosine Matrix
  Subtract : Sum  Inputs=+-
  SunAngle : Scope
  unitVector : Subsystem
  Sun Angle : Outport
  S_hat : Outport  Port=2
  wires:
  Spacecraft Position/1 -> Subtract/2  "r_sat"
  Planetary Ephemeris/1 -> Subtract/1  "r_sun"
  julian_date/1 -> Planetary Ephemeris/1
  Subtract/1 -> Product1/2  "r_satsun"
  Dot Product/1 -> Acos/1
  Acos/1 -> SunAngle/1, Sun Angle/1
  q_icrf2b/1 -> Quaternions to Direction Cosine Matrix1/1
  Quaternions to Direction Cosine Matrix1/1 -> Product1/1  "icrf2b"
  Product1/1 -> unitVector/1(X)  "S_body"
  Normal/1 -> Dot Product/1
  unitVector/1(X_hat) -> Dot Product/2, Gain/1  "-S_hat"
  Gain/1 -> S_hat/1

== system SolarSail/icrf2lvlh ==
  quat_icrf : Inport
  pos_icrf : Inport  Port=2
  vel_icrf : Inport  Port=3
  DCM_icrf2lvlh : Subsystem
  Direction Cosine Matrix to Quaternions : sharedtransform/Direction Cosine Matrix  to Quaternions  aMode=0  action=Warning  tolerance=eps(4)
      settings: LibrarySourceBlock=|
      | aerolibtransform2/Direction Cosine Matrix
      | to Quaternions
  Quaternion Multiplication : aerolibutil/Quaternion Multiplication
  quat_lvlh : Outport
  wires:
  quat_icrf/1 -> Quaternion Multiplication/2
  Direction Cosine Matrix to Quaternions/1 -> Quaternion Multiplication/1
  Quaternion Multiplication/1 -> quat_lvlh/1
  DCM_icrf2lvlh/1(DCM) -> Direction Cosine Matrix to Quaternions/1
  pos_icrf/1 -> DCM_icrf2lvlh/1(pos)
  vel_icrf/1 -> DCM_icrf2lvlh/2(vel)

== system SolarSail/pos2altitude ==
  pos : Inport
  Dot Product : DotProduct  OutDataTypeStr=Inherit: Inherit via internal rule
  R_earth : Constant  Value=6371000
  Square Root : Sqrt
  Subtract : Sum  Inputs=+-
  Altitude : Outport
  wires:
  pos/1 -> Dot Product/2, Dot Product/1
  Dot Product/1 -> Square Root/1
  Square Root/1 -> Subtract/1  "Radius"
  R_earth/1 -> Subtract/2
  Subtract/1 -> Altitude/1

== system SolarSail/Atmospheric Drag/Drag Angle ==
  v : Inport
  Acos : Trigonometry  Operator=acos
  Constant : Constant  Value=[0;0;1]
  Dot Product : DotProduct  OutDataTypeStr=Inherit: Inherit via internal rule
  unitVector : Subsystem
  unitVector1 : Subsystem
  dragAngle : Outport
  wires:
  v/1 -> unitVector/1(X)
  Constant/1 -> unitVector1/1(X)
  unitVector/1(X_hat) -> Dot Product/1  "v_hat"
  unitVector1/1(X_hat) -> Dot Product/2  "N_hat"
  Dot Product/1 -> Acos/1
  Acos/1 -> dragAngle/1

== system SolarSail/Atmospheric Drag/unitVector ==
  X : Inport
  Divide : Product  Inputs=*/
  Dot Product : DotProduct  OutDataTypeStr=Inherit: Inherit via internal rule
  Square Root : Sqrt
  X_hat : Outport
  wires:
  X/1 -> Divide/1, Dot Product/2, Dot Product/1
  Dot Product/1 -> Square Root/1
  Square Root/1 -> Divide/2
  Divide/1 -> X_hat/1

== system SolarSail/Atmospheric Drag/v_atm ==
  pos : Inport
  latitude : Inport  Port=2
  Cos : Trigonometry  Operator=cos
  Cross Product : matrix_library/Cross Product
  Degrees to Radians : simulink_extras/Transformations/Degrees to Radians
  Divide : Product  Inputs=**
  Earth Angular Vel : Constant  Value=2*pi/86400
  Multiply1 : Gain  Gain=[0;0;1]
  v_atm : Outport
  wires:
  pos/1 -> Cross Product/2
  latitude/1 -> Degrees to Radians/1
  Cos/1 -> Divide/2
  Divide/1 -> Multiply1/1
  Multiply1/1 -> Cross Product/1  "rotational velocity"
  Cross Product/1 -> v_atm/1
  Degrees to Radians/1 -> Cos/1
  Earth Angular Vel/1 -> Divide/1

== system SolarSail/Atmospheric Drag/v_icrf2v_body ==
  q : Inport
  v : Inport  Port=2
  Matrix Multiply : Product  Multiplication=Matrix(*)
  Quaternions to Direction Cosine Matrix : sharedtransform/Quaternions to  Direction Cosine Matrix  aMode=aMode
      settings: LibrarySourceBlock=|
      | aerolibtransform2/Quaternions to
      | Direction Cosine Matrix
  v_body : Outport
  wires:
  q/1 -> Quaternions to Direction Cosine Matrix/1
  Quaternions to Direction Cosine Matrix/1 -> Matrix Multiply/1
  v/1 -> Matrix Multiply/2
  Matrix Multiply/1 -> v_body/1

== system SolarSail/CubeSat Animation/Antenna Position to VRML ==
  x : Inport
  ECEF to VRML : Subsystem
  Length Conversion : aerolibconvert2/Length Conversion  IU=m  OU=km
  km to VRML units : Gain  Gain=1/1000
  xVRML : Outport  VectorParamsAs1DForOutWhenUnconnected=off
  wires:
  Length Conversion/1 -> km to VRML units/1
  km to VRML units/1 -> ECEF to VRML/1(M)
  x/1 -> Length Conversion/1
  ECEF to VRML/1(VR) -> xVRML/1

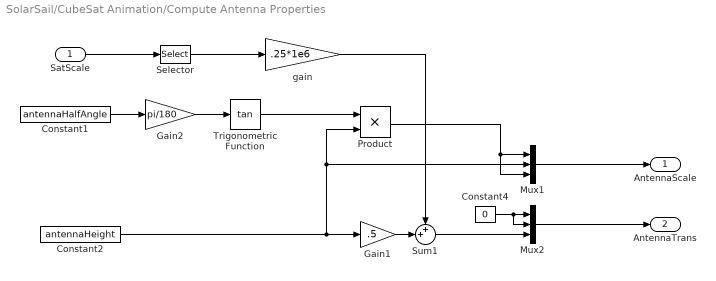
== system SolarSail/CubeSat Animation/Compute Antenna Properties ==
  SatScale : Inport
  Constant1 : Constant  Value=antennaHalfAngle
  Constant2 : Constant  Value=antennaHeight
  Constant4 : Constant  Value=0
  Gain1 : Gain  Gain=.5
  Gain2 : Gain  Gain=pi/180
  Mux1 : Mux  Inputs=3
  Mux2 : Mux  Inputs=3
  Product : Product
  Selector : Selector  InputPortWidth=3  IndexOptions=Index vector (dialog)  Indices=1  OutputSizes=1
  Sum1 : Sum  Inputs=++|
  Trigonometric Function : Trigonometry  Operator=tan
  gain : Gain  Gain=.25*1e6
  AntennaScale : Outport  VectorParamsAs1DForOutWhenUnconnected=off
  AntennaTrans : Outport  Port=2  VectorParamsAs1DForOutWhenUnconnected=off
  wires:
  Gain2/1 -> Trigonometric Function/1
  Constant4/1 -> Mux2/1, Mux2/2
  Sum1/1 -> Mux2/3
  Constant2/1 -> Gain1/1, Mux1/2, Product/2
  gain/1 -> Sum1/1
  Constant1/1 -> Gain2/1
  Product/1 -> Mux1/3, Mux1/1
  Gain1/1 -> Sum1/2
  Trigonometric Function/1 -> Product/1
  Mux2/1 -> AntennaTrans/1
  Mux1/1 -> AntennaScale/1
  SatScale/1 -> Selector/1
  Selector/1 -> gain/1

== system SolarSail/CubeSat Animation/Compute Earth Rotation Rate ==
  EarthRot : Inport
  Constant : Constant  Value=0
  Constant1 : Constant  Value=0
  Euler Angles to Quaternions : aerolibobsolete/Euler Angles to Quaternions
  Quaternion to VRML : Subsystem
  Sum : Sum  Inputs=|++
  Unit Delay : UnitDelay  SampleTime=-1  HasFrameUpgradeWarning=on
  Vector Concatenate : Concatenate  NumInputs=3
  VRMLRot : Outport  VectorParamsAs1DForOutWhenUnconnected=off
  wires:
  Quaternion to VRML/1(AxisAngle) -> VRMLRot/1
  Euler Angles to Quaternions/1 -> Quaternion to VRML/1(q)
  Vector Concatenate/1 -> Euler Angles to Quaternions/1
  Constant1/1 -> Vector Concatenate/2
  Constant/1 -> Vector Concatenate/1
  Sum/1 -> Unit Delay/1, Vector Concatenate/3
  Unit Delay/1 -> Sum/2
  EarthRot/1 -> Sum/1

== system SolarSail/CubeSat Animation/Compute Umbra Translation ==
  I : Inport
  Add : Sum
  ConeHalfLength : Gain  Gain=692
  InvertSunPosECEF : Gain  Gain=-1
  unitVec : Subsystem
  O : Outport  VectorParamsAs1DForOutWhenUnconnected=off
  wires:
  ConeHalfLength/1 -> Add/2
  I/1 -> InvertSunPosECEF/1
  Add/1 -> O/1
  InvertSunPosECEF/1 -> unitVec/1(I), Add/1
  unitVec/1(O) -> ConeHalfLength/1

== system SolarSail/CubeSat Animation/Quaternion to VRML ==
  q : Inport
  Demux : Demux
  "Flip 180 deg, rotate 90" : Constant  Value=[0 -.7071 .7071 0]
  Gain : Gain  Gain=2
  Mux : Mux
  Quaternion Multiplication : aerolibutil/Quaternion Multiplication
  Selector : Selector  InputPortWidth=4  IndexOptions=Index vector (dialog)  Indices=[3 4 2 1]  OutputSizes=1
  Trigonometric Function : Trigonometry  Operator=acos
  axis_angle : Outport  VectorParamsAs1DForOutWhenUnconnected=off
  wires:
  Demux/4 -> Mux/4
  Demux/3 -> Mux/3
  Demux/2 -> Mux/2
  Gain/1 -> Mux/1
  Selector/1 -> axis_angle/1
  q/1 -> Quaternion Multiplication/1
  Mux/1 -> Selector/1
  Trigonometric Function/1 -> Gain/1
  Demux/1 -> Trigonometric Function/1
  "Flip 180 deg, rotate 90"/1 -> Quaternion Multiplication/2
  Quaternion Multiplication/1 -> Demux/1

== system SolarSail/CubeSat Animation/Quaternion to VRML1 ==
  q : Inport
  Demux : Demux
  "Flip 180 deg, rotate 90" : Constant  Value=[0 -0.7071 0.7071 0]
  Gain : Gain  Gain=2
  Mux : Mux
  Quaternion Multiplication : aerolibutil/Quaternion Multiplication
  Selector : Selector  InputPortWidth=4  IndexOptions=Index vector (dialog)  Indices=[3 4 2 1]  OutputSizes=1
  Trigonometric Function : Trigonometry  Operator=acos
  axis_angle : Outport  VectorParamsAs1DForOutWhenUnconnected=off
  wires:
  Demux/4 -> Mux/4
  Demux/3 -> Mux/3
  Demux/2 -> Mux/2
  Gain/1 -> Mux/1
  Selector/1 -> axis_angle/1
  Mux/1 -> Selector/1
  Trigonometric Function/1 -> Gain/1
  Demux/1 -> Trigonometric Function/1
  "Flip 180 deg, rotate 90"/1 -> Quaternion Multiplication/2
  q/1 -> Quaternion Multiplication/1
  Quaternion Multiplication/1 -> Demux/1

== system SolarSail/CubeSat Animation/Radar on//off ==
  NavMode : Inport
  Add : Sum  Inputs=-+
  Compare To Constant : simulink/Logic and Bit Operations/Compare To Constant  relop===  const=1  OutDataTypeStr=boolean  ZeroCross=off
  Constant : Constant
  Data Type Conversion : DataTypeConversion  OutDataTypeStr=double  SaturateOnIntegerOverflow=off  RndMeth=Floor
  Gain : Gain  Gain=0.6
  Radar : Outport  VectorParamsAs1DForOutWhenUnconnected=off
  wires:
  NavMode/1 -> Compare To Constant/1
  Compare To Constant/1 -> Data Type Conversion/1
  Data Type Conversion/1 -> Gain/1
  Gain/1 -> Add/1
  Constant/1 -> Add/2
  Add/1 -> Radar/1

== system SolarSail/CubeSat Animation/Sat Position to VRML ==
  x : Inport
  ECEF to VRML : Subsystem
  Length Conversion : aerolibconvert2/Length Conversion  IU=m  OU=km
  km to VRML units : Gain  Gain=1/1000
  xVRML : Outport  VectorParamsAs1DForOutWhenUnconnected=off
  wires:
  ECEF to VRML/1(VR) -> xVRML/1
  x/1 -> Length Conversion/1
  km to VRML units/1 -> ECEF to VRML/1(M)
  Length Conversion/1 -> km to VRML units/1

== system SolarSail/CubeSat Animation/Satellite Model Scaling ==
  Constant : Constant  Value=cubesatSize
  Mux : Mux  Inputs=3
  ScaleModelToVRML : Gain  Gain=1/.3e6
  Out1 : Outport  VectorParamsAs1DForOutWhenUnconnected=off
  wires:
  ScaleModelToVRML/1 -> Mux/3, Mux/1, Mux/2
  Constant/1 -> ScaleModelToVRML/1
  Mux/1 -> Out1/1

== system SolarSail/CubeSat Animation/Sun Position to VRML ==
  x : Inport
  ECEF to VRML : Subsystem
  Length Conversion : aerolibconvert2/Length Conversion  IU=m  OU=km
  km to VRML units : Gain  Gain=1/1000
  xVRML : Outport  VectorParamsAs1DForOutWhenUnconnected=off
  wires:
  ECEF to VRML/1(VR) -> xVRML/1
  x/1 -> Length Conversion/1
  km to VRML units/1 -> ECEF to VRML/1(M)
  Length Conversion/1 -> km to VRML units/1

== system SolarSail/Desired Position/If Action Subsystem ==
  In1 : Inport
  In2 : Inport  Port=2
  Action Port : ActionPort  ActionPortLabel=case [ 0 ]:
  des1_lvlh : Outport
  des2_lvlh : Outport  Port=2
  wires:
  In1/1 -> des1_lvlh/1
  In2/1 -> des2_lvlh/1

== system SolarSail/Desired Position/If Action Subsystem1 ==
  In1 : Inport
  In2 : Inport  Port=2
  Action Port : ActionPort  ActionPortLabel=case [ 1 ]:
  des1_lvlh : Outport
  des1_lvlh1 : Outport  Port=2
  wires:
  In1/1 -> des1_lvlh/1
  In2/1 -> des1_lvlh1/1

== system SolarSail/Disturbance Torques/Atmospheric Drag Torque ==
  F_drag : Inport
  Cross Product : matrix_library/Cross Product
  Scope : Scope
  c_p : Constant  Value=[0;0;-0.15]
  T : Outport
  wires:
  Cross Product/1 -> T/1, Scope/1
  c_p/1 -> Cross Product/1
  F_drag/1 -> Cross Product/2

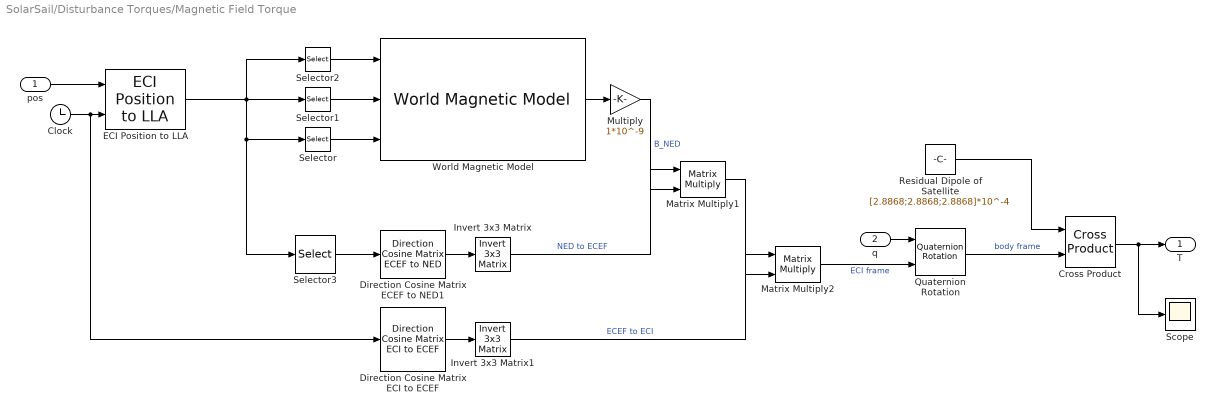
== system SolarSail/Disturbance Torques/Magnetic Field Torque ==
  pos : Inport
  q : Inport  Port=2
  Clock : Clock
  Cross Product : matrix_library/Cross Product
  Direction Cosine Matrix ECEF to NED1 : aerolibtransform2/Direction Cosine Matrix ECEF to NED
  Direction Cosine Matrix ECI to ECEF : aerolibtransform2/Direction Cosine Matrix ECI to ECEF  red=IAU-2000/2006  year=2024  month=July  day=11  hour=2  min=0  sec=0  deltaT=Sec  errorflag=Error  extraparamflag=off
      settings: AttributesFormatString=%<red>
  ECI Position to LLA : aerolibtransform2/ECI Position to LLA  red=IAU-2000/2006  year=2024  month=July  day=11  hour=2  min=0  sec=0  deltaT=Sec  errorflag=Error  extraparamflag=off  eunits=Metric (MKS)  earthmodel=WGS84  flat=1/298.257223563  eqradius=6378137
      settings: AttributesFormatString=%<red>
  Invert 3x3 Matrix : aerolibutil/Invert  3x3 Matrix
  Invert 3x3 Matrix1 : aerolibutil/Invert  3x3 Matrix
  Matrix Multiply1 : Product  Multiplication=Matrix(*)
  Matrix Multiply2 : Product  Multiplication=Matrix(*)
  Multiply : Gain  Gain=1*10^-9
  Quaternion Rotation : aerolibutil/Quaternion Rotation
  Residual Dipole of Satellite : Constant  Value=[2.8868;2.8868;2.8868]*10^-4
  Scope : Scope
  Selector : Selector  InputPortWidth=3  IndexOptions=Index vector (dialog)  Indices=[2]  OutputSizes=1
  Selector1 : Selector  InputPortWidth=3  IndexOptions=Index vector (dialog)  Indices=[1]  OutputSizes=1
  Selector2 : Selector  InputPortWidth=3  IndexOptions=Index vector (dialog)  Indices=[3]  OutputSizes=1
  Selector3 : Selector  InputPortWidth=3  IndexOptions=Index vector (dialog)  Indices=[1 2]  OutputSizes=1
  World Magnetic Model : aerolibgravity2/World Magnetic Model  model=WMM2020 (2020-2025)  customFile='WMM2020.COF'  units=Metric (MKS)  time_in=off  month=July  day=11  year=2024  action=Error  h_out=off  dec_out=off  inc_out=off  ti_out=off
  T : Outport
  wires:
  Clock/1 -> Direction Cosine Matrix ECI to ECEF/1, ECI Position to LLA/2
  pos/1 -> ECI Position to LLA/1
  Selector/1 -> World Magnetic Model/3
  Selector1/1 -> World Magnetic Model/2
  ECI Position to LLA/1 -> Selector3/1, Selector/1, Selector2/1, Selector1/1
  Selector2/1 -> World Magnetic Model/1
  World Magnetic Model/1 -> Multiply/1
  Selector3/1 -> Direction Cosine Matrix ECEF to NED1/1
  Direction Cosine Matrix ECEF to NED1/1 -> Invert 3x3 Matrix/1
  Direction Cosine Matrix ECI to ECEF/1 -> Invert 3x3 Matrix1/1
  Invert 3x3 Matrix/1 -> Matrix Multiply1/1  "NED to ECEF"
  Invert 3x3 Matrix1/1 -> Matrix Multiply2/1  "ECEF to ECI"
  Matrix Multiply1/1 -> Matrix Multiply2/2
  Matrix Multiply2/1 -> Quaternion Rotation/2  "ECI frame"
  q/1 -> Quaternion Rotation/1
  Quaternion Rotation/1 -> Cross Product/2  "body frame"
  Multiply/1 -> Matrix Multiply1/2  "B_NED"
  Residual Dipole of Satellite/1 -> Cross Product/1
  Cross Product/1 -> Scope/1, T/1

== system SolarSail/Disturbance Torques/SRP Torque ==
  F_srp : Inport
  Cross Product : matrix_library/Cross Product
  Scope : Scope
  c_p : Constant  Value=[0.01;0.01;-0.15]
  T : Outport
  wires:
  Cross Product/1 -> T/1, Scope/1
  c_p/1 -> Cross Product/1
  F_srp/1 -> Cross Product/2

== system SolarSail/RCDs/Absorption Force ==
  SRP : Inport
  Area : Inport  Port=2
  SunAngle : Inport  Port=3
  Cos : Trigonometry  Operator=cos
  F_sun : Subsystem
  Product : Product
  Abs Force : Outport
  wires:
  SRP/1 -> F_sun/1(SRP)
  SunAngle/1 -> Cos/1, F_sun/3(sun angle)
  Area/1 -> F_sun/2(area)
  Product/1 -> Abs Force/1
  F_sun/1(F_sun) -> Product/1
  Cos/1 -> Product/2

== system SolarSail/RCDs/Diffusive Force ==
  SRP : Inport
  Area : Inport  Port=2
  SunAngle : Inport  Port=3
  Add : Sum
  Cos : Trigonometry  Operator=cos
  F_normal : Subsystem
  F_sun : Subsystem
  Product : Product
  Diff Force : Outport
  wires:
  F_sun/1(F_sun) -> Product/1
  F_normal/1(F_normal) -> Add/1
  Add/1 -> Diff Force/1
  SRP/1 -> F_normal/1(SRP), F_sun/1(SRP)
  SunAngle/1 -> Cos/1, F_sun/3(sun angle), F_normal/3(sun angle)
  Area/1 -> F_sun/2(area), F_normal/2(area)
  Cos/1 -> Product/2
  Product/1 -> Add/2

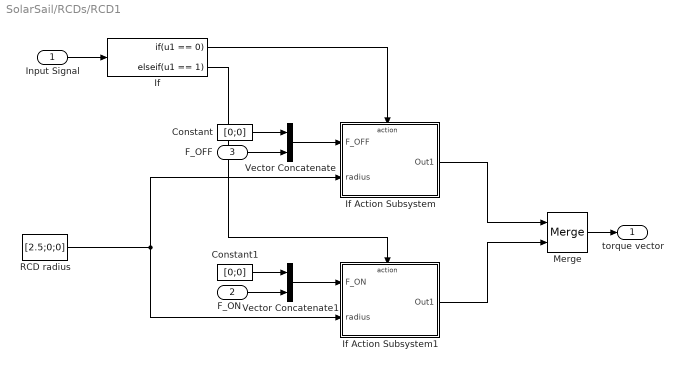
== system SolarSail/RCDs/RCD1 ==
  Input Signal : Inport
  F_ON : Inport  Port=2
  F_OFF : Inport  Port=3
  Constant : Constant  Value=[0;0]
  Constant1 : Constant  Value=[0;0]
  If : If  IfExpression=u1 == 0  ElseIfExpressions=u1 == 1  ShowElse=off
  If Action Subsystem : Subsystem  TreatAsAtomicUnit=on
  If Action Subsystem1 : Subsystem  TreatAsAtomicUnit=on
  Merge : Merge
  RCD radius : Constant  Value=[2.5;0;0]
  Vector Concatenate : Concatenate
  Vector Concatenate1 : Concatenate
  torque vector : Outport
  wires:
  Input Signal/1 -> If/1
  If/1 -> If Action Subsystem/Action
  Merge/1 -> torque vector/1
  If Action Subsystem/1(Out1) -> Merge/1
  If/2 -> If Action Subsystem1/Action
  If Action Subsystem1/1(Out1) -> Merge/2
  RCD radius/1 -> If Action Subsystem/2(radius), If Action Subsystem1/2(radius)
  Vector Concatenate/1 -> If Action Subsystem/1(F_OFF)
  Constant/1 -> Vector Concatenate/1
  F_OFF/1 -> Vector Concatenate/2
  F_ON/1 -> Vector Concatenate1/2
  Constant1/1 -> Vector Concatenate1/1
  Vector Concatenate1/1 -> If Action Subsystem1/1(F_ON)

== system SolarSail/RCDs/RCD2 ==
  Input Signal : Inport
  F_ON : Inport  Port=2
  F_OFF : Inport  Port=3
  Constant : Constant  Value=[0;0]
  Constant1 : Constant  Value=[0;0]
  If : If  IfExpression=u1 == 0  ElseIfExpressions=u1 == 1  ShowElse=off
  If Action Subsystem : Subsystem  TreatAsAtomicUnit=on
  If Action Subsystem1 : Subsystem  TreatAsAtomicUnit=on
  Merge : Merge
  RCD radius : Constant  Value=[0;2.5;0]
  Vector Concatenate : Concatenate
  Vector Concatenate1 : Concatenate
  torque vector : Outport
  wires:
  Input Signal/1 -> If/1
  If/1 -> If Action Subsystem/Action
  Merge/1 -> torque vector/1
  If Action Subsystem/1(Out1) -> Merge/1
  If/2 -> If Action Subsystem1/Action
  If Action Subsystem1/1(Out1) -> Merge/2
  RCD radius/1 -> If Action Subsystem/2(radius), If Action Subsystem1/2(radius)
  Vector Concatenate/1 -> If Action Subsystem/1(F_OFF)
  Constant/1 -> Vector Concatenate/1
  F_OFF/1 -> Vector Concatenate/2
  F_ON/1 -> Vector Concatenate1/2
  Constant1/1 -> Vector Concatenate1/1
  Vector Concatenate1/1 -> If Action Subsystem1/1(F_ON)

== system SolarSail/RCDs/RCD3 ==
  Input Signal : Inport
  F_ON : Inport  Port=2
  F_OFF : Inport  Port=3
  Constant : Constant  Value=[0;0]
  Constant1 : Constant  Value=[0;0]
  If : If  IfExpression=u1 == 0  ElseIfExpressions=u1 == 1  ShowElse=off
  If Action Subsystem : Subsystem  TreatAsAtomicUnit=on
  If Action Subsystem1 : Subsystem  TreatAsAtomicUnit=on
  Merge : Merge
  RCD radius : Constant  Value=[-2.5;0;0]
  Vector Concatenate : Concatenate
  Vector Concatenate1 : Concatenate
  torque vector : Outport
  wires:
  Input Signal/1 -> If/1
  If/1 -> If Action Subsystem/Action
  Merge/1 -> torque vector/1
  If Action Subsystem/1(Out1) -> Merge/1
  If/2 -> If Action Subsystem1/Action
  If Action Subsystem1/1(Out1) -> Merge/2
  RCD radius/1 -> If Action Subsystem/2(radius), If Action Subsystem1/2(radius)
  Vector Concatenate/1 -> If Action Subsystem/1(F_OFF)
  Constant/1 -> Vector Concatenate/1
  F_OFF/1 -> Vector Concatenate/2
  F_ON/1 -> Vector Concatenate1/2
  Constant1/1 -> Vector Concatenate1/1
  Vector Concatenate1/1 -> If Action Subsystem1/1(F_ON)
